simulink model "ornek_6_2"  (R2023b)
settings: Solver=FixedStepDiscrete  StartTime=0.0  StopTime=10  FixedStep=0.1  RelTol=1e-3  EnableMultiTasking=on
undefined symbols (not defined in the file): Timer
libraries: MCHP_Blockset x5, simulink_extras x1
settings Model: Creator=bugra  LastModifiedBy=bugra
settings OptimizationCC: DefaultParameterBehavior=Inlined  DefaultUnderspecifiedDataType=single  EnhancedBackFolding=on  BooleansAsBitfields=on  PassReuseOutputArgsAs=Individual arguments  ZeroExternalMemoryAtStartup=off  ZeroInternalMemoryAtStartup=off  OptimizeBlockOrder=speed  DifferentSizesBufferReuse=on  EfficientTunableParamExpr=on
settings DebuggingCC: ParameterTunabilityLossMsg=error
settings HardwareCC: ProdBitPerInt=16  ProdBitPerPointer=16  ProdBitPerSizeT=16  ProdBitPerPtrDiffT=32  ProdLargestAtomicInteger=Integer  ProdLargestAtomicFloat=None  ProdWordSize=16  ProdHWDeviceType=Generic->Custom
settings ModelReferenceCC: ModelReferenceNumInstancesAllowed=Single
settings SFSimCC: MATLABDynamicMemAlloc=off
settings RTWCC: Description=Microchip Embedded Target PIC24 dsPIC30 dsPIC33 (real-time)  SystemTargetFile=MCHP_dsPIC_stf.tlc  TemplateMakefile=MCHP_dsPIC.tmf
settings CodeAppCC: ForceParamTrailComments=on  IgnoreCustomStorageClasses=off  MaxIdLength=255  OperatorAnnotations=on  SimulinkDataObjDesc=on  SFDataObjDesc=on  InsertBlockDesc=on
settings STFCustomTargetCC: TargetLibSuffix=_lib.a  MultiwordLength=256  CombineOutputUpdateFcns=on  CombineSignalStateStructs=on  SuppressErrorStatus=on  ERTCustomFileBanners=on  SupportContinuousTime=off  RemoveResetFunc=on  MATLABClassNameForMDSCustomization=Simulink.SoftwareTarget.ERTCustomization  SystemTargetFile=MCHP_dsPIC_stf.tlc
settings ERTTargetCC: TargetLibSuffix=_lib.a  TargetLangStandard=C99 (ISO)  ParMdlRefBuildCompliant=off  CompOptLevelCompliant=off  ConcurrentExecutionCompliant=off  CombineSignalStateStructs=on  SuppressErrorStatus=on  SupportNonInlinedSFcns=on  ModelStepFunctionPrototypeControlCompliant=off  CPPClassGenCompliant=off  UseToolchainInfoCompliant=off  ExtModeStaticAllocSize=500  InlinedParameterPlacement=NonHierarchical  ERTSrcFileBannerTemplate=MCHP_dsPIC_code_template.cgt  ERTHdrFileBannerTemplate=MCHP_dsPIC_code_template.cgt  ERTDataSrcFileTemplate=MCHP_dsPIC_code_template.cgt  ERTDataHdrFileTemplate=MCHP_dsPIC_code_template.cgt  ERTCustomFileTemplate=MCHP_main.tlc  MaxLineWidth=110

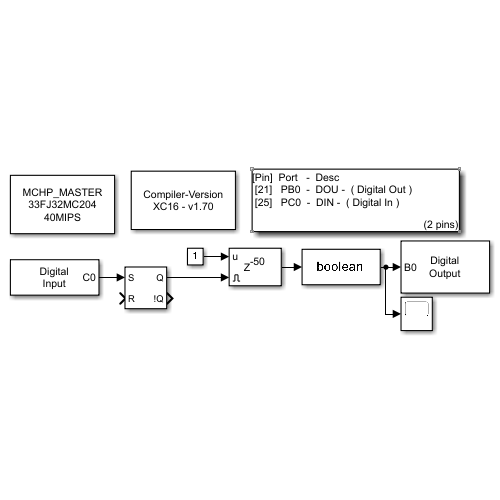
[thumbnail: Simulink's stored preview of the top-level diagram]
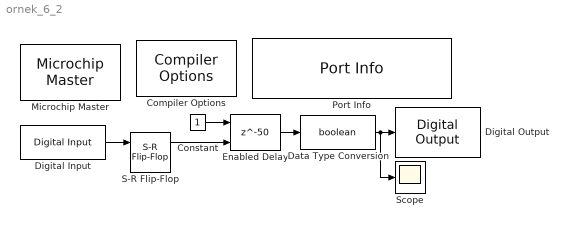
== system ornek_6_2 ==
  Compiler Options : MCHP_Blockset/System Configuration/Compiler Options  Priority=1  LATEST_CMPLR=off  COMP_LIST_TXT=XC16 - v1.70  DFP_LIST_TXT=v 1.4.235  CMSIS_DSP_TXT=Dynamic Options  USE_64BIT_DOUBLE=off  MCHP_MULTITHREAD_COMPILATION=on  UseCustom_LinkerScript=off  MCHP_MASTERLINK=ornek_6_2/Microchip Master  OPTIMIZATION_LEVEL=2  MPLAB_LINKLIB=default  MPLAB_LINKLIB1=fast floating-point math  CodeReplacement_TXT=None  OPTIMIZATION_FLTO=off  OPTIMIZATION_REORDER=off  OPTIMIZATION_ASM_REORDER=off  UNROLL_LOOPS=off  PROCEDURAL_ABSTRACTION=off  GC_SECTIONS=None  MCODE=is less than 32768 (faster)  MCONST=in data memory  MDATA=Use only memory below address 8192 (faster)  MSCALAR=Use only memory below address 8192 (faster)  MLARGEARRAY=off  MAGGREGATE=off  HEAP_SIZE=0  OMF=elf  DEBUG_INFO=off  MCHP_STACK_USAGE=off  GCC_STACK_USAGE=off  ProduceHexOutput=on  AssemblyListing=off  SaveTemps=off  NO_EDS_WARN=on  PRINT_STATISTICS=off
      settings: SourceProductName=MPLAB Device Blocks for Simulink
  Constant : Constant
  Data Type Conversion : DataTypeConversion  OutDataTypeStr=boolean  SaturateOnIntegerOverflow=off  RndMeth=Floor
  Digital Input : MCHP_Blockset/Digital IO/Digital Input  PORT_TXT="C   [ 0 : 9 ]"  PIN=[0]  INPUT_PIN_MODE=Hi-impedance (default)  PACK=off  SIMULTANEOUS=off  ORDERING=None  SampleTime=-1  MCHP_PORT={Digital In}{DIN}2:0:C0;  MCHP_MASTERLINK=ornek_6_2/Microchip Master
      settings: SourceProductName=MPLAB Device Blocks for Simulink
  Digital Output : MCHP_Blockset/Digital IO/Digital Output  PORT=Dynamic Options  PORT_TXT="B   [ 0 : 15 ]"  PIN=0  INIT_VALUE=-1  PACK=off  OUTPUT_PIN_MODE=Push-Pull (default)  SIMULTANEOUS=off  READPREVIOUS=off  ORDERING=None  SampleTime=-1  MCHP_MASTERLINK=ornek_6_2/Microchip Master
      settings: SourceProductName=MPLAB Device Blocks for Simulink
  Enabled Delay : Delay  DelayLength=50  ShowEnablePort=on
      settings: InputPortMap=u0,e6
  Microchip Master : MCHP_Blockset/System Configuration/Microchip Master  Priority=1  PICREF=33FJ32MC204  TIMESTEP_REF="Timer  ( 0.1s )"  BUSYFLAG=Dynamic Options  BUSYFLAG_TXT=None  VDD_range=Dynamic Options  PWRTEN=Not used  BOREN=Enabled  BODENV=2.7V  BORV=Not used  FPWRT=128ms  DSBOREN=Disable ZPBOR during Deep Sleep Mode  DSLPBOR=Not used  MCLRE=Enabled  SMCLR=MCLR pin generates a normal system Reset  PMDL1WAY=Allow only one reconfiguration  RSTPRI=Device will obtain reset instruction from Primary flash  TEMP=Not used  SOSCSRC=Not used  SOSCSEL=Not used  IOL1WAY=Allow Only One Re-configuration  ALTVREF=Not used  DISUVREG=Not used  DSSWEN=Not used  LPCFG=Not used  RTCBAT=Not used  VBTBOR=Not used  WUTSEL=Not used  POWERSAVE=off  FNOSC=Primary Oscillator (XT; HS; EC)  FPR=ECIO w/ PLL 16x  FOSFPR=HS3 w/PLL 16x  FOS=Primary Oscillator  FRANGE=High Range  OSCILLATOR_SELECT=Crystal / Ceramic resonator  OSCILLATOR_SELECT_spd=Crystal / Ceramic resonator  QUARTZ=10e6  QUARTZ_spd=10e6  POSCGAIN=2x gain setting  POSCBOOST=Boost the kick start of the oscillator  SOSCGAIN=2x gain setting  SOSCBOOST=Boost the kick start of the oscillator  ACTIV_PLL=on  ACTIV_PLL_spd=on  MIPS_DESIRED=40000000  MIPS_DESIRED_spd=40000000  CPUDIV=Divide by 1  FPLLMUL=Not used  FPLLIDIV=8x Divider  POSCFREQ=Not used  POSCMD=HS Oscillator Mode  POSCMOD=Primary osc disabled  MIPS=40 * 1e6  ACLKCON=Optimized for PWM resolution & ADC conversion speed  ACLKCON_spd=Optimized for PWM resolution & ADC conversion speed  FPLLODIV=32x Divider  PLLKEN=Clock switch to PLL source will wait until the PLL lock signal is valid  FCKSM=Clock switching is enabled; Fail-Safe Clock Monitor is Disabled  FCKSMEN=Sw Disabled; Mon Disabled  IESO=Start up with FRC; then switch  DSWDTPS=1:2^36  FWDTEN=Disable  FWDTWINSZ=Window size is 25%  FWPSA=1:512  FWPSA0=1:128  FWPSB=1:16  WDT=Disable  WDTPOST=1:32768  WDTPRE=1:128  WDTPS=1:1048576  WINDIS=Watchdog Timer in Non-Window mode  WWDTEN=Window mode  DSWDTEN=Disable DSWDT during Deep Sleep Mode  DSWDTOSC=Select LPRC as DSWDT Reference clock  FWDT_RCLKSEL=WDT Run Mode uses BFRC:256  FWDT_RWDTPS=1:2147483648  FWDT_SWDTMPS=1:2147483648  FWDT_WDTEN=Enable  FWDT_WDTRSTEN=WDT event generates a reset  FWDT_WDTWIN=WDT Window is 25% of WDT period  FWDT_WINEN=Not used  FPBDIV=Not used  FSOSCEN=Disable Secondary Oscillator  LPRCSEL=Not used  OSCIOFCN=Not used  OSCIOFNC=general purpose digital I/O pin  LVRCFG=Not used  PLL_96MHZ=Not used  PLL96MHZ=Not used  PLLDIV=Not used  WDTCLK=Not used  WDTCMX=Not used  WDTWIN=Watchdog Window is 25% of WDT period  XTCFG=24-32 MHz crystals  XTBST=Boost the kick-start  APL=Aux Flash Code protect is disabled  APLK=Aux Flash Write Protection or Code Protection is Enabled  AWRP=Auxiliary program memory is not write-protected  BSS=No Boot program Flash segment  BWP=Not used  BWRP=Boot Segment may be written  CP=Protection Disabled  EBS=No Boot EEPROM  ESS=No Segment Data EEPROM  GCP=General Segment Code protect is Disabled  GSS=High Security Code Protection Enabled  GSS0=Not used  GSSK=General Segment Write Protection or Code Protection is Enabled  GWRP=General Segment may be written  PWP=Not used  RBS=No Boot RAM  RSS=No Secure RAM  SSS=No Secure Segment  SWRP=Secure segment may be written  WPCFG=Not used  WPDIS=Not used  WPEND=Not used  WPFP=Not used  ICESEL=Communicate on PGEC1/PGED1  ICS=Communicate on PGEC1 and PGED1  JTAGEN=Disable  FICD_JTAGEN=Disable  COE=Not used  RES=Not used  DEBUG=Debugger is disabled  BACKBUG=Not used  BKBUG=Not used  ALTI2C=I2C mapped to SDA1/SCL1 pins  ALTI2C1=SDA1/SCK1 pins are selected as the I/O pins for I2C1  ALTI2C2=SDA2/SCK2 pins are selected as the I/O pins for I2C2  ALTI2C3=I2C3 mapped to SDA3/SCL3 pins  FDEVOPT1_ALTI2C1=Not used  FDEVOPT1_ALTI2C2=Not used  FDEVOPT1_SPI2MAPDIS=Not used  FDEVOPT_ALTI2C1=Primary I2C1 pins are used  FDEVOPT_ALTI2C2=Primary I2C2 pins are used  FDEVOPT_ALTI2C3=Primary I2C3 pins are used  FDEVOPT_SPI2PIN=SPI2 pins are selected by peripheral pin selection feature  ALTQIO=QEA1; QEB1; INDX1 are selected as inputs to QEI1  ALTSS1=SS1A is selected as the I/O pin for SPI1  CMPPOL0=Hysteresis is applied to falling edge  CMPPOL1=Hysteresis is applied to falling edge  FCANIO=Not used  FETHIO=Default Ethernet I/O  FMIIEN=MII Enabled  FSRSSEL=Not used  FUSBIDIO=Controlled by the USB Module  FVBUSONIO=Not used  HPOL=PWM module high side output pins have active-high output polarity  HYST0=45 mV Hysteresis  HYST1=45 mV Hysteresis  I2C1SEL=Not used  LPOL=PWM module low side output pins have active-high output polarity  PWMPIN=PWM module pins controlled by PORT register at device Reset  RTCOSC=Not used  UPLLEN=USB PLL Disabled  UPLLIDIV=Not used  ATMOD8=Not used  ALTPMP=Not used  I2C2SEL=Not used  ALTADREF=Not used  ALTCVREF=Not used  PWMLOCK=PWM registers may be written without key sequence  INT_PRIORITY_DMA=0  MCHP_TIMER_REQUEST={Time Step}{TS}0:2:3:1:[]:4000000;  MCHP_TIMER_RESULT=[1 62498.999999999992724 ]  MCHP_PLLRegisters="[5    110  16385     -1     -1]"  MCHPVAR=MCHP.fcy.MIPS=40000000;MCHP.fcy.SYSCLK=40000000;MCHP.fcy.ADC=40000000;MCHP.fcy.Comparator=40000000;MCHP.fcy.I2C=40000000;MCHP.fcy.SPI=40000000;MCHP.fcy.UART=40000000;MCHP.fcy.Timers=40000000;MCHP.fcy.OC=40000000;MCHP.fcy.IC=40000000;MCHP.fcy.Ports=40000000;MCHP.fcy.QEI=40000000;MCHP.PowerSave=0;MCHP.TimeStepFactor=MCHP_Fun.Hex2num('3FF0000000000001');MCHP.TimeStep_Timer=1;MCHP.NTIMERS=3;MCHP.id.name='33FJ32MC204';MCHP.id.N=reshape([33 32 204],1,3);MCHP.id.L=reshape({ 'FJ','MC',''},1,3);MCHP.id.Arch=3;MCHP.id.maskset='';MCHP.id.dos='00899';MCHP.id.ds='70000283';MCHP.id.archTxt='33xxxx';MCHP.id.clonedfrom='DSPIC33FJ32MC204';MCHP.id.isSlave=0;MCHP.id.isMaster=0;MCHP.periph.PPS.reg_RPINRx=reshape([-1 1 1 -1 -1 -1 1 1 -1 -1 -1 -1 -1 -1 1 1 -1 -1 -1 -1 1 1 -1 -1 1 -1 1 -1 1 1 1 -1 -1 -1 -1 -1 1 1 -1 -1 1 1 1],1,43);MCHP.periph.pin.ODCx=reshape([1951 65535 1023 0 0 0 0 0 0 0 0],1,11);MCHP.PPS.dsPIC.RP=reshape([16 17 18 19 20 21 22 23 24 25 26 27 28 29 30 31 32 33 34 35 36 37 38 39 40 41],1,26);MCHP.PPS.dsPIC.RPI=[];MCHP.PPS.dsPIC.RPINR_list=reshape({ '1','INT1','INT2','INT3','INT4','T1CK','T2CK','T3CK','T4CK','T5CK','T6CK','T7CK','T8CK','T9CK','IC1','IC2','IC3','IC4','IC5','IC6','IC7','IC8','OCFA','OCFB','FLT1','FLT2','FLT3','FLT4','QEIA1','QEIB1','QEINDX1','QEIHOM1','QEIA2','QEIB2','QEINDX2','QEIHOM2','U1RX','U1CTS','U2RX','U2CTS','SDI1','SCK1_in','SS1_in','44','SDI2','SCK2_in','SS2_in','48','CSDIR','CSCK','COFS','52','C1RX','C2RX','U3RX','U3CTS','U4RX','U4CTS','SDI3','SCK3_in','SS3_in','62','SDI4','SCK4_in','SS4_in','66','IC9','IC10','IC11','IC12','IC13','IC14','IC15','IC16','OCFC','SYNCI1','SYNCI2','DTCMP1','DTCMP2','DTCMP3','DTCMP4','DTCMP5','DTCMP6','DTCMP7','FLT5','FLT6','FLT7','FLT8','89','SENT1','SENT2','92'},1,92);MCHP.PPS.dsPIC.RPOR_list=reshape({ '1','C1OUT','C2OUT','U1TX','U1RTS','U2TX','U2RTS','SDO1','SCK1_out','SS1_out','SDO2','SCK2_out','SS2_out','CSDO','CSCK','COFS','C1TX','17','OC1','OC2','OC3','OC4','22','23','24','25','UPDN1','UPDN2'},1,28);MCHP.PPS.dsPIC.RPV=reshape([-1 -1 -1 -1 -1 -1],1,6);MCHP.PPS.map_RPnR_RPORx=reshape([0 1 2 3 4 5 6 7 8 9 10 11 12 13 14 15 16 17 18 19 20 21 22 23 24 25],1,26);MCHP.Rx=reshape([19 21 25 -1 -1 -1 -1 -1 -1 -1 -1 20 22 26 -1 -1 -1 -1 -1 -1 -1 -1 30 23 27 -1 -1 -1 -1 -1 -1 -1 -1 31 24 36 -1 -1 -1 -1 -1 -1 -1 -1 34 33 37 -1 -1 -1 -1 -1 -1 -1 -1 -1 41 38 -1 -1 -1 -1 -1 -1 -1 -1 -1 42 2 -1 -1 -1 -1 -1 -1 -1 -1 13 43 3 -1 -1 -1 -1 -1 -1 -1 -1 32 44 4 -1 -1 -1 -1 -1 -1 -1 -1 35 1 5 -1 -1 -1 -1 -1 -1 -1 -1 12 8 -1 -1 -1 -1 -1 -1 -1 -1 -1 -1 9 -1 -1 -1 -1 -1 -1 -1 -1 -1 -1 10 -1 -1 -1 -1 -1 -1 -1 -1 -1 -1 11 -1 -1 -1 -1 -1 -1 -1 -1 -1 -1 14 -1 -1 -1 -1 -1 -1 -1 -1 -1 -1 15 -1 -1 -1 -1 -1 -1 -1 -1 -1],11,16);MCHP.ADC.ANtype=reshape([3 0],1,2);MCHP.ADC.ADCONx=reshape([59375 59327 40959 0 0 0],1,6);MCHP.ADC.ADCHS_0=reshape([40863 1799],1,2);MCHP.ADC.Flags=reshape([1 0],1,2);MCHP.ADC.Buffer=reshape([16 -1],1,2);MCHP.ADC.port=reshape([0 1 16 17 18 19 32 33 34 -1 -1 -1 -1 -1 -1 -1 -1 -1 -1 -1 -1 -1 -1 -1 -1 -1 -1 -1 -1 -1 -1 -1 -1 -1 -1 -1 -1 -1 -1 -1 -1 -1 -1 -1 -1 -1 -1 -1 -1 -1 -1 -1 -1 -1 -1 -1 -1],1,57);MCHP.ADC.port_ALT=reshape([-1 -1 -1 -1],1,4);MCHP.ADC.port_ALTA=reshape([-1 -1 -1 -1],1,4);MCHP.ADC.port_ALTB=reshape([-1 -1 -1 -1],1,4);MCHP.ADC.port_ALTC=reshape([-1 -1 -1 -1],1,4);MCHP.ADC.port_VrefP=0;MCHP.ADC.port_VrefM=1;MCHP.ADC.port_AVdd=-1;MCHP.ADC.port_AVss=-1;MCHP.ADC.ADCDATA=reshape([0 0 0 0 0 0 0 0 0 0 0 0 0 0 0 0 0 0 0 0 0 0 0 0 0 0 0 0 0 0 0 0 0 0 0 0 0 0 0 0 0 0 0 0 0 0 0 0 0 0 0 0 0 0 0 0 0],1,57);MCHP.ADC.HS_SAR.TRGSRC=reshape([0 0 0 0 0 0 0 0 0 0 0 0 0 0 0 0 0 0 0 0 0 0 0 0 0 0 0 0 0 0 0 0],1,32);MCHP.ADC.HS_SAR.nFilters=0;MCHP.ADC.HS_SAR.nDedicatedCore=0;MCHP.ADC.HS_SAR.CALIBRATION=0;MCHP.ADC.HS_SAR.ADCON1L=-1;MCHP.ADC.HS_SAR.ADC_Class3_idxStart=32;MCHP.memory.RAM=2048;MCHP.memory.RAM_XBegin=2048;MCHP.memory.RAM_YBegin=3072;MCHP.memory.RAM_dma=reshape([-1 -1],1,2);MCHP.memory.FLASH_ECC=0;MCHP.DMA.Num=0;MCHP.DMA.CNTmax=0;MCHP.QEI.QEICONx=reshape([49151 -1 -1 -1 -1 -1],1,6);MCHP.QEI.QEItype=1;MCHP.QEI.Port_QEI_INDX=reshape([-1 -1],1,2);MCHP.QEI.Port_QEI_QEA=reshape([-1 -1],1,2);MCHP.QEI.Port_QEI_QEB=reshape([-1 -1],1,2);MCHP.QEI.Port_QEI_UPDN=reshape([-1 -1],1,2);MCHP.INT.Port=reshape([23 32767 32767 -1 -1],1,5);MCHP.ADC1.port=reshape([-1 -1 -1 -1 -1 -1 -1 -1 -1 -1 -1 -1 -1 -1 -1 -1 -1 -1 -1 -1 -1 -1 -1 -1 -1 -1 -1 -1 -1 -1 -1 -1],1,32);MCHP.ADC2.port=reshape([-1 -1 -1 -1 -1 -1 -1 -1 -1 -1 -1 -1 -1 -1 -1 -1 -1 -1 -1 -1 -1 -1 -1 -1 -1 -1 -1 -1 -1 -1 -1 -1],1,32);MCHP.ADC3.port=reshape([-1 -1 -1 -1 -1 -1 -1 -1 -1 -1 -1 -1 -1 -1 -1 -1],1,16);MCHP.ADC4.port=reshape([-1 -1 -1 -1 -1 -1 -1 -1 -1 -1 -1 -1 -1 -1 -1 -1],1,16);MCHP.ADC5.port=reshape([-1 -1 -1 -1 -1 -1 -1 -1 -1 -1 -1 -1 -1 -1 -1 -1],1,16);MCHP.ADC1N.port=reshape([-1 -1 -1 -1],1,4);MCHP.ADC2N.port=reshape([-1 -1 -1 -1],1,4);MCHP.ADC3N.port=reshape([-1 -1 -1 -1],1,4);MCHP.ADC4N.port=reshape([-1 -1 -1 -1],1,4);MCHP.ADC5N.port=reshape([-1 -1 -1 -1],1,4);MCHP.PWM_HS.Flags=reshape([0 0 0],1,3);MCHP.PWM.port_FLT=reshape([-1 -1 -1 -1 -1 -1 -1 -1 -1 -1 -1 -1 -1 -1 -1 -1 -1 -1 -1 -1 -1 -1 -1 -1 -1 -1 -1 -1 -1 -1 -1 -1 -1],1,33);MCHP.PWM.PWMRef=2;MCHP.PWM.Flag=2;MCHP.PWM.Port_PWM_l=reshape([31 39 29 -1 27 -1 -1 -1 -1 -1 -1 -1 -1 -1 -1 -1 -1 -1 -1 -1 -1 -1 -1 -1],2,12);MCHP.PWM.Port_PWM_h=reshape([30 38 28 -1 26 -1 -1 -1 -1 -1 -1 -1 -1 -1 -1 -1 -1 -1 -1 -1 -1 -1 -1 -1],2,12);MCHP.PWM_HS_FEP.nEVTOUT=-1;MCHP.IC.Port=reshape([32767 32767 0 0 0 0 32767 32767 0 0 0 0 0 0 0 0],1,16);MCHP.IC.type=0;MCHP.OC.Port=reshape([32767 32767 0 0 0 0 32767 32767 0 0 0 0 0 0 0 0],1,16);MCHP.OC.type=0;MCHP.CN.Port=reshape([4 20 0 1 16 17 18 19 32 33 34 31 30 29 28 27 26 39 38 41 40 25 24 23 22 36 37 21 35 3 2 -1 -1 -1 -1 -1 -1 -1 -1 -1 -1 -1 -1 -1 -1 -1 -1 -1 -1 -1 -1 -1 -1 -1 -1 -1 -1 -1 -1 -1 -1 -1 -1 -1 -1 -1 -1 -1 -1 -1 -1 -1 -1 -1 -1 -1 -1 -1 -1 -1 -1 -1 -1 -1 -1],1,85);MCHP.CN.PullUp=reshape([65535 32767 0 0 0 0 0 0 0 0 0],1,11);MCHP.CN.type=0;MCHP.CN.Flag_PullDown=1;MCHP.SPI.Refs=reshape([1 0 0 0 0 0],1,6);MCHP.SPI.SPIxCON1=8191;MCHP.SPI.SPIxCON2=57346;MCHP.SPI.SPIxFIFOSIZE=-1;MCHP.SPI.Port_SDI=reshape([-1 -1 -1 -1 -1 -1],1,6);MCHP.SPI.Port_SDO=reshape([-1 -1 -1 -1 -1 -1],1,6);MCHP.SPI.Port_SCK=reshape([-1 -1 -1 -1 -1 -1],1,6);MCHP.SPI.Port_SS=reshape([-1 -1 -1 -1 -1 -1],1,6);MCHP.I2C.Refs=reshape([1 0 0 0 0],1,5);MCHP.I2C.I2CxCON=65535;MCHP.I2C.NewRegName=1;MCHP.I2C.Port_SDA=reshape([25 -1 -1 -1 -1],1,5);MCHP.I2C.Port_SCL=reshape([24 -1 -1 -1 -1],1,5);MCHP.I2C.Port_ASDA=reshape([21 -1 -1 -1 -1],1,5);MCHP.I2C.Port_ASCL=reshape([22 -1 -1 -1 -1],1,5);MCHP.I2C.Fuse_Port_SCL_SDA=reshape([16 1 -1 -1 -1 -1 -1 -1 -1 -1],2,5);MCHP.I2C.Fuse_Port_ASCL_ASDA=reshape([16 2 -1 -1 -1 -1 -1 -1 -1 -1],2,5);MCHP.SCCP.nSCCP=0;MCHP.SCCP.MCCP=reshape([0 0 0 0 0 0 0 0 0],1,9);MCHP.PGA.Port_PGA1P=reshape([-1 -1 -1 -1],1,4);MCHP.PGA.Port_PGA1N=reshape([-1 -1 -1 -1],1,4);MCHP.PGA.Port_PGA2P=reshape([-1 -1 -1 -1],1,4);MCHP.PGA.Port_PGA2N=reshape([-1 -1 -1 -1],1,4);MCHP.PGA.Num=0;MCHP.HS_AnalogComparator.Port_CMP1=reshape([-1 -1 -1 -1],1,4);MCHP.HS_AnalogComparator.Port_CMP2=reshape([-1 -1 -1 -1],1,4);MCHP.HS_AnalogComparator.Port_CMP3=reshape([-1 -1 -1 -1],1,4);MCHP.HS_AnalogComparator.Port_CMP4=reshape([-1 -1 -1 -1],1,4);MCHP.HS_AnalogComparator.Port_CMP5=reshape([-1 -1 -1 -1],1,4);MCHP.HS_AnalogComparator.Port_CMP6=reshape([-1 -1 -1 -1],1,4);MCHP.HS_AnalogComparator.Port_EXTREFx=reshape([-1 -1],1,2);MCHP.HS_AnalogComparator.Port_DACOUTx=reshape([-1 -1],1,2);MCHP.HS_AnalogComparator.Num=0;MCHP.Comp.Port_CVrefin=-1;MCHP.Comp.Port_CVref=-1;MCHP.Comp.Port_CVref1O=-1;MCHP.Comp.Port_CVref2O=-1;MCHP.Comp.Port_CxOUT=reshape([32767 32767 32767 32767 32767],1,5);MCHP.Comp.Port_OAxOUT=reshape([-1 -1 -1 -1 -1],1,5);MCHP.Comp.Port_CxINP=reshape([-1 17 -1 -1 -1],1,5);MCHP.Comp.Port_CxINM=reshape([-1 -1 -1 -1 16 -1 -1 -1 -1 -1 -1 -1 -1 -1 -1 -1 -1 -1 -1 -1],4,5);MCHP.Comp.Port_OAxINP=reshape([-1 -1 -1 -1 -1],1,5);MCHP.Comp.Port_OAxINM=reshape([-1 -1 -1 -1 -1],1,5);MCHP.Comp.nComp=reshape([5 0 0],1,3);MCHP.Comp.OpAmp=0;MCHP.Comp.CVRCON=reshape([0 0],1,2);MCHP.Comp.CMCON=0;MCHP.CDAC.Port_DACx=reshape([-1 -1 -1],1,3);MCHP.CDAC.nCDAC=0;MCHP.UART.port_Rx=reshape([32767 -1 -1 -1 -1 -1],1,6);MCHP.UART.port_Tx=reshape([32767 -1 -1 -1 -1 -1],1,6);MCHP.UART.port_ARx=reshape([-1 -1],1,2);MCHP.UART.port_ATx=reshape([-1 -1],1,2);MCHP.UART.port_RTS=reshape([32767 -1 -1 -1 -1 -1],1,6);MCHP.UART.port_CTS=reshape([32767 -1 -1 -1 -1 -1],1,6);MCHP.UART.reg_UxMODE=reshape([48127 -1 -1 -1 -1 -1],1,6);MCHP.UART.reg_UxSTA=reshape([61439 -1 -1 -1 -1 -1],1,6);MCHP.modsrc.DOS_04094_cpu_33a_v1_dspic33a=0;MCHP.modsrc.DOS_04436_perseus_dspic33a=0;MCHP.modsrc.DOS_04928_gpio_ports_upb_v2_dspic33a=0;MCHP.modsrc.DOS_02672_math_progcrc_upb_v1_dspic33a=0;MCHP.modsrc.DOS_04993_sec_32bit_cp_upb_v1_dspic33a=0;MCHP.modsrc.DOS_03681_bmx_33a_upb_v1_dspic33a=0;MCHP.modsrc.DOS_03459_adc_pc_ctrl_upb_v2_dspic33a=0;MCHP.modsrc.DOS_04302_pwm_pc_upb_v3_dspic33a=0;MCHP.modsrc.DOS_03076_uart_protocol_upb_v1_dspic33a=0;MCHP.modsrc.DOS_01482_spi_i2s_upb_v1_dspic33a=0;MCHP.modsrc.DOS_05155_i2c_upb_v4_dspic33a=0;MCHP.modsrc.DOS_02359_sent_j2716_upb_v1_dspic33a=0;MCHP.modsrc.DOS_05177_qei_32b_upb_v2_dspic33a=0;MCHP.modsrc.DOS_01512_ccp_mccp_upb_v1_dspic33a=0;MCHP.modsrc.DOS_03496_dac_pdm_nbit_upb_v2_dspic33a=0;MCHP.modsrc.DOS_02673_tmr_classa_upb_v1_dspic33a=0;MCHP.modsrc.DOS_04776_perf_mon_upb_v1_dspic33a=0;MCHP.modsrc.DOS_03680_pfm_pbu_33a_upb_v1_dspic33a=0;MCHP.modsrc.DOS_04649_sec_pac_upb_v0_dspic33a=0;MCHP.modsrc.DOS_03966_io_integrity_monitor_upb_v1_dspic33a=0;MCHP.modsrc.DOS_04641_biss_master_upb_v1_dspic33a=0;MCHP.modsrc.DOS_04077_dma_upb_v1_dspic33a=0;MCHP.modsrc.DOS_04549_nvm_ctrl_32bit_upb_v1_dspic33a=0;MCHP.modsrc.DOS_04449_clk_cru_33a_upb_v1_dspic33a=0;MCHP.modsrc.DOS_03850_clk_monitor_upb_v1_dspic33a=0;MCHP.modsrc.DOS_04342_osc_rc8mhz_ctrl_upb_v4_dspic33a=0;MCHP.modsrc.DOS_04650_wdt_upb_v4_dspic33a=0;MCHP.modsrc.DOS_05178_ptg_pc_upb_v1_dspic33a=0;MCHP.modsrc.DOS_04181_data_ram_ctrl_upb_v1_dspic33a=0;MCHP.modsrc.DOS_04735_wdt_dmt_upb_v6_dspic33a=0;MCHP.modsrc.DOS_01577_cla_clc_upb_v1_dspic33a=0;MCHP.modsrc.DOS_03516_pwr_sib_upb_v3_dspic33a=0;MCHP.modsrc.DOS_03495_amp_pad_opamp_ctrl_upb_v2_dspic33a=0;MCHP.modsrc.DOS_05308_pegasus_dspic33a=0;MCHP.modsrc.DOS_02976_adc_12b_upb_v2_dspic33a=0;MCHP.modsrc.DOS_05404_adc_pc_ctrl_upb_v3_dspic33a=0;MCHP.modsrc.DOS_05226_pwm_pc_upb_v4_dspic33a=0;MCHP.modsrc.DOS_05226_apwm_pc_upb_v4_dspic33a=0;MCHP.modsrc.DOS_05431_dac_pdm_nbit_upb_v3_dspic33a=0;MCHP.modsrc.DOS_04649_sec_pac_upb_v1_dspic33a=0;MCHP.modsrc.DOS_05461_pwr_sib_upb_v4_dspic33a=0;MCHP.modsrc.DOS_05420_amp_vref_ctl_upb_v1_dspic33a=0;MCHP.modsrc.DOS_03267_adc_soft_code_seq_v1_dspic33a=0;MCHP.modsrc.DOS_04537_can_fd_upb_v3_dspic33a=0;MCHP.modsrc.DOS_05346_sec_cam_lite_v2_dspic33a=0;MCHP.modsrc.DOS_05830_blueRidge_dspic33a=0;MCHP.modsrc.DOS_05765_math_rdc_upb_v1_32bit=0;MCHP.modsrc.DOS_05908_math_cic_upb_v2_32bit=0;MCHP.modsrc.DOS_05922_i3c_upb_v1_32bit=0;MCHP.modsrc.DOS_05442_icd_trace_33a_v1_dspic33a=0;MCHP.modsrc.DOS_02551_cpu_16bit_v7=0;MCHP.modsrc.DOS_01520_wdt_dmt_upb_v1_16bit=0;MCHP.modsrc.DOS_02359a_sent_j2716_upb_v1=0;MCHP.modsrc.DOS_02672_math_progcrc_upb_v1_16bit=0;MCHP.modsrc.DOS_01577_cla_clc_upb_v1=0;MCHP.modsrc.DOS_02915_ecc_v2=0;MCHP.modsrc.DOS_02673_tmr_classa_upb_v1_16bit=0;MCHP.modsrc.DOS_01494_qei_32b_upb_v1_16bit=0;MCHP.modsrc.DOS_02472_ppi_pmp16_upb_v1_16bit=0;MCHP.modsrc.DOS_01441_i2c_upb_v1_16bit_TLAH=0;MCHP.modsrc.DOS_03076_uart_protocol_upb_v1_16bit=0;MCHP.modsrc.DOS_01482=0;MCHP.modsrc.DOS_01483_pwm_16bit=0;MCHP.modsrc.DOS_02949_WACG=0;MCHP.modsrc.DOS_02316_nvm_ctrl_v1_16bit=0;MCHP.modsrc.DOS_03349_amp_pad_opamp_ctrl_upb_v1=0;MCHP.modsrc.DOS_02653_afe_current_bias_ctrl_upb_v1_16bit=0;MCHP.modsrc.DOS_01459_ptg_pc_upb_v1_16bit=0;MCHP.modsrc.DOS_01512_ccp_mccp_upb_v1_16bit=0;MCHP.modsrc.DOS_02519_dma_sfr_16bit_v2=0;MCHP.modsrc.DOS_02508c11=0;MCHP.modsrc.DOS_02475_dac_pdm_nbit_upb_v1_16bit=0;MCHP.modsrc.DOS_02467_gpio_upb_v1_16bit=0;MCHP.modsrc.DOS_00805_rst_integration_v4=0;MCHP.modsrc.DOS_02659_clk_sib_v12=0;MCHP.modsrc.DOS_02237_osc_dco_ctrl_upb_v1_16bit=0;MCHP.modsrc.DOS_02674_wdt_upb_v1_16bit=0;MCHP.modsrc.DOS_01407=0;MCHP.modsrc.DOS_03247_CAN_FD_UPB_V2_16_bit=0;MCHP.modsrc.DOS_03994_WAC07=0;MCHP.modsrc.DOS_02552_msi_upb_v1_Master=0;MCHP.modsrc.DOS_03667_pwm_pc_upb_v2_16bit=0;MCHP.modsrc.DOS_04180_drm_ctrl_ecc_v1=0;MCHP.modsrc.DOS_03431_STX03=0;MCHP.modsrc.DOS_03516_pwr_sib_upb_v3=0;MCHP.modsrc.DOS_02552_msi_upb_v1_Slave=0;MCHP.modsrc.DOS_04621_amp_pga_ctrl_upb_v3=0;MCHP.modsrc.DOS_02497_WACV=0;MCHP.modsrc.DOS_02593_amp_pga_ctrl_pb_v2_16bit=0;MCHP.modsrc.DOS_01461_afe_ctmu_con_upb_v1_16bit=0;MCHP.modsrc.DOS_02497_WACA=0;MCHP.modsrc.DOS_02478_uart_irda_upb_v1_16bit=0;MCHP.modsrc.DOS_00929=0;MCHP.modsrc.DOS_01198=0;MCHP.modsrc.DOS_03029_WACH=0;MCHP.modsrc.DOS_01483_apwm_16bit=0;MCHP.modsrc.DOS_04797_WAC0A=0;MCHP.modsrc.DOS_04884_WAC0B=0;MCHP.modsrc.DOS_04797_WAC09=0;MCHP.modsrc.DOS_03662_WACU=0;MCHP.modsrc.DOS_00794=0;MCHP.modsrc.DOS_00931=0;MCHP.modsrc.DOS_00932=0;MCHP.modsrc.DOS_00942=0;MCHP.modsrc.DOS_00938=0;MCHP.modsrc.DOS_00996=0;MCHP.modsrc.DOS_00997=0;MCHP.modsrc.DOS_00998=0;MCHP.modsrc.DOS_00209=0;MCHP.modsrc.DOS_01555_adc=0;MCHP.modsrc.DOS_01293=0;MCHP.modsrc.DOS_00828=0;MCHP.modsrc.DOS_01116=0;MCHP.modsrc.DOS_01017_RPORx=0;MCHP.modsrc.DOS_01017_RPINRx=0;MCHP.modsrc.DOS_01555_nvm_tsmc18_v2_16bit=0;MCHP.modsrc.DOS_00804=0;MCHP.modsrc.DOS_00826=0;MCHP.modsrc.DOS_01555_TLAK_PMDx=0;MCHP.modsrc.DOS_01555_TLAK_INT_=0;MCHP.modsrc.DOS_00933=0;MCHP.modsrc.DOS_01555=0;MCHP.modsrc.DOS_01555_ptg=0;MCHP.modsrc.DOS_00958=0;MCHP.modsrc.DOS_01117_PORTx=0;MCHP.modsrc.DOS_00999=0;MCHP.modsrc.DOS_01041=0;MCHP.modsrc.DOS_00892=0;MCHP.modsrc.DOS_01287_TLAC_PMDx=0;MCHP.modsrc.DOS_01287_TLAC_INT_=0;MCHP.modsrc.DOS_01424=0;MCHP.modsrc.DOS_01332=0;MCHP.modsrc.DOS_01468_PMBA_current_source=0;MCHP.modsrc.DOS_02291_PGA=0;MCHP.modsrc.DOS_01467_Comparator=0;MCHP.modsrc.DOS_01498_TLAY=0;MCHP.modsrc.DOS_00993_PLL_120MHz=0;MCHP.modsrc.DOS_01332_ptg_pc_v1=0;MCHP.modsrc.DOS_00958_pwm_TLAY=0;MCHP.modsrc.TLAY_IOPorts=0;MCHP.modsrc.DOS_00929q=0;MCHP.modsrc.DOS_02415_spi_v5=0;MCHP.modsrc.DOS_RPINRx_16bit_2=0;MCHP.modsrc.DOS_01497_TLAH_PMDx=0;MCHP.modsrc.DOS_02550_TLAL_INT=0;MCHP.modsrc.DOS_00958_pwm_TLAH=0;MCHP.modsrc.DOS_01287_TLAH_INT_=0;MCHP.modsrc.DOS_01113=0;MCHP.modsrc.DOS_01017_PMDx=0;MCHP.modsrc.DOS_00927=0;MCHP.modsrc.DOS_01080=0;MCHP.modsrc.DOS_00794_cpu_16bit_v3=0;MCHP.modsrc.DOS_02192_TLCD_PMDx=0;MCHP.modsrc.DOS_02192_TLCD_INT_=0;MCHP.modsrc.DOS_02192_cmp=0;MCHP.modsrc.DOS_00958_pwm_TLCD=0;MCHP.modsrc.DOS_02192_PORTx_TLCD=0;MCHP.modsrc.DOS_00936=0;MCHP.modsrc.DOS_00995=0;MCHP.modsrc.DOS_00546=0;MCHP.modsrc.DOS_00474=0;MCHP.modsrc.DOS_02481_WACK_MC_Config=0;MCHP.modsrc.DOS_03088_pfm_cache_ocp_v2_WACK=0;MCHP.modsrc.DOS_02819_pfm_ctrl_32bit_upb_v2=0;MCHP.modsrc.DOS_02674_wdt_upb_v1_32bit=0;MCHP.modsrc.DOS_01520_wdt_dmt_upb_v1=0;MCHP.modsrc.DOS_02869_icd_jtag_bvci_upb_v2=0;MCHP.modsrc.DOS_02823_WACJ_clk_cru_upb_v2=0;MCHP.modsrc.DOS_02823_WACN_clk_cru_upb_v2=0;MCHP.modsrc.DOS_01423_RPINRx=0;MCHP.modsrc.DOS_02481_RPORx=0;MCHP.modsrc.DOS_02511_pwr_sib_upb_v1_32bit=0;MCHP.modsrc.DOS_02907_WACN_GP_int_evic_v3=0;MCHP.modsrc.DOS_01500_dma_bvci_v2=0;MCHP.modsrc.DOS_02141_tmr_classa_pb_v2=0;MCHP.modsrc.DOS_02815_tmr_classb_upb_v1=0;MCHP.modsrc.DOS_00740_icap_pb_v1=0;MCHP.modsrc.DOS_00749_ocmp_pb_v1=0;MCHP.modsrc.DOS_01441_i2c_upb_v1_32bit=0;MCHP.modsrc.DOS_01329_spi_pb_v2=0;MCHP.modsrc.DOS_02478_uart_irda_upb_v1_32bit=0;MCHP.modsrc.DOS_03554_cmp_control_upb_v2_32bit=0;MCHP.modsrc.DOS_01445_dac_nbit__control_upb_v1_32bit=0;MCHP.modsrc.DOS_01461_afe_ctmu_con_upb_v1=0;MCHP.modsrc.DOS_01577_cla_clc_upb_v1_32bit=0;MCHP.modsrc.DOS_02467_gpio_ports_upb_v1=0;MCHP.modsrc.DOS_02508_adc_sar_ctrl_upb_v1_PIC32MK=0;MCHP.modsrc.DOS_01261_tmr_rtcc_pb_v2=0;MCHP.modsrc.DOS_01475_lpwr_deep_sleep_ctrl_v2=0;MCHP.modsrc.DOS_EIP_00136_ssx_v1=0;MCHP.modsrc.DOS_02907_WACN_MC_int_evic_v3=0;MCHP.modsrc.DOS_01477_pwm_mc_upb_v1=0;MCHP.modsrc.DOS_01494_qei_32b_upb_v1=0;MCHP.modsrc.DOS_03247_can_fd_upb_v2_pic32mk=0;MCHP.modsrc.DOS_02907_WACK_MC_int_evic_v3=0;MCHP.modsrc.DOS_02514_dfm_strl_sst_upb_v1=0;MCHP.modsrc.DOS_02472_ppi_pmp16_upb_v1=0;MCHP.modsrc.DOS_02813a_usb_otgcore_pb_v3=0;MCHP.modsrc.DOS_02481_WACJ_MC_Config=0;MCHP.modsrc.DOS_02569_pfm_cache_ocp_v1=0;MCHP.modsrc.DOS_02481_WACJ_MC_int_evic_v3=0;MCHP.modsrc.DOS_01459_ptg_pc_upb_v1_SIC=0;MCHP.modsrc.DOS_01427_cmp_control_upb_v1_32bit=0;MCHP.modsrc.DOS_01152_can_bvci_v1=0;MCHP.modsrc.DOS_02787_WACD_Config=0;MCHP.modsrc.DOS_00800_dac_4bit_ctrl_pb_v1=0;MCHP.modsrc.DOS_01539_icd_jtag_pb_v2=0;MCHP.modsrc.DOS_02823_clk_cru_upb_v2=0;MCHP.modsrc.DOS_01423_RPORx=0;MCHP.modsrc.DOS_02907_WACD_int_evic_v3=0;MCHP.modsrc.DOS_00734_uart_irda_pb_v1=0;MCHP.modsrc.DOS_00687_tmr_classa_pb_v1=0;MCHP.modsrc.DOS_00745_tmr_classb_pb_v1=0;MCHP.modsrc.DOS_02508_adc_sar_ctrl_upb_v1=0;MCHP.modsrc.DOS_00866_cmp_control_pb_v2=0;MCHP.modsrc.DOS_01114_eth_bvci_v1=0;MCHP.modsrc.DOS_02831_usb_clk_rst_v2=0;MCHP.modsrc.DOS_01643_pfm_cache_ahb_v2=0;MCHP.modsrc.DOS_EIP_00206r5_sqi_v2=0;MCHP.modsrc.DOS_EIP_00124_usb_hs_otgcore_v1=0;MCHP.modsrc.DOS_EIP_00218_math_rng_ahbs_v2=0;MCHP.modsrc.DOS_EIP_00109_ebi_v1=0;MCHP.modsrc.DOS_EIP_00158_crypto_v1=0;MCHP.PortBase=16;MCHP.PortPrefixe='P';MCHP.clock.PBxDIV=-1;MCHP.clock.CLKx_INTDIV=reshape([-1 -1 -1 -1 -1 -1 -1 -1 -1 -1 -1 -1 -1],1,13);MCHP.clock.CLKx_FRACDIV=reshape([-1 -1 -1 -1 -1 -1 -1 -1 -1 -1 -1 -1 -1],1,13);  MCHP_CRC=20034748  BTMODE=Device is in Single Boot (legacy) mode  RES1=Not used  PLLSS=Not used  RES2=Not used  ALTCMPI=Not used  BOREN1=Not used  ALTRB6=Not used  RETCFG=Not used  DFMCY=Not used  BSS2=No Boot Segment  BSEN=No Boot Segment  CWRP=Configuration Segment may be written  CSS=No Protection (other than CWRP)  AIVTDIS=Disable Alternate Vector Table  BSLIM=Not used  WDTEN=Disable  BTSWP=BOOTSWP instruction is disabled  DBCC=No Cross Connection between DAC outputs  CTXT1=Not Assigned  CTXT2=Not Assigned  SEQNUM=Not used  nSEQNUM=Not used  BOREN0=Enabled  DMTIVT=Not used  DMTCNT=2^8 (256)  DMTEN=Dead Man Timer is Disabled and can be enabled by software  ON=Not used  USERID=Not used  RESERVED1=Not used  PGL1WAY=Allow only one reconfiguration  FPLLRNG=34-68 MHz Input  FPLLICLK=FRC is input to the System PLL  FPLLMULT=PLL Multiply by 128  UPLLFSEL=USB PLL input is 24 MHz  DMTINTV=Window/Interval value is 127/128 counter value  WDTSPGM=WDT stops during Flash programming  FDMTEN=Deadman Timer is disabled  TRCEN=Trace features in the CPU are enabled  BOOTISA=Boot code and Exception code is MIPS32  FECCCON=ECC and Dynamic ECC are disabled (ECCCON bits are writable)  EXTDDRSIZE=Not used  FSLEEP=Flash is powered down when the device is in Sleep mode  DBGPER=Allow CPU access to all permission regions  EJTAGBEN=Normal EJTAG functionality  TSEQ=Not used  CSEQ=Not used  RWDTPS=1:1048576  RCLKSEL=Always use LPRC  SWDTPS=1:1048576  DMTIVTL=Not used  DMTIVTH=Not used  DMTCNTL=Not used  DMTCNTH=Not used  DMTDIS=Dead Man Timer is Disabled and can be enabled by software  SMBEN=SMBus input threshold is enabled  SPI2PIN=SPI2 uses I/O remap (PPS) pins  CTXT3=Not Assigned  CTXT4=Not Assigned  MBXM0=Mailbox register configured for Main data read (Secondary to Main data transfer)  MBXM1=Mailbox register configured for Main data read (Secondary to Main data transfer)  MBXM2=Mailbox register configured for Main data read (Secondary to Main data transfer)  MBXM3=Mailbox register configured for Main data read (Secondary to Main data transfer)  MBXM4=Mailbox register configured for Main data read (Secondary to Main data transfer)  MBXM5=Mailbox register configured for Main data read (Secondary to Main data transfer)  MBXM6=Mailbox register configured for Main data read (Secondary to Main data transfer)  MBXM7=Mailbox register configured for Main data read (Secondary to Main data transfer)  MBXM8=Mailbox register configured for Main data read (Secondary to Main data transfer)  MBXM9=Mailbox register configured for Main data read (Secondary to Main data transfer)  MBXM10=Mailbox register configured for Main data read (Secondary to Main data transfer)  MBXM11=Mailbox register configured for Main data read (Secondary to Main data transfer)  MBXM12=Mailbox register configured for Main data read (Secondary to Main data transfer)  MBXM13=Mailbox register configured for Main data read (Secondary to Main data transfer)  MBXM14=Mailbox register configured for Main data read (Secondary to Main data transfer)  MBXM15=Mailbox register configured for Main data read (Secondary to Main data transfer)  MBXHSA=MSIxMBXD15 assigned to mailbox handshake protocol block A  MBXHSB=MSIxMBXD15 assigned to mailbox handshake protocol block B  MBXHSC=MSIxMBXD15 assigned to mailbox handshake protocol block C  MBXHSD=MSIxMBXD15 assigned to mailbox handshake protocol block D  MBXHSE=MSIxMBXD15 assigned to mailbox handshake protocol block E  MBXHSF=MSIxMBXD15 assigned to mailbox handshake protocol block F  MBXHSG=MSIxMBXD15 assigned to mailbox handshake protocol block G  MBXHSH=MSIxMBXD15 assigned to mailbox handshake protocol block H  HSAEN=Mailbox data flow control handshake protocol block disabled  HSBEN=Mailbox data flow control handshake protocol block disabled  HSCEN=Mailbox data flow control handshake protocol block disabled  HSDEN=Mailbox data flow control handshake protocol block disabled  HSEEN=Mailbox data flow control handshake protocol block disabled  HSFEN=Mailbox data flow control handshake protocol block disabled  HSGEN=Mailbox data flow control handshake protocol block disabled  HSHEN=Mailbox data flow control handshake protocol block disabled  CPRA0=Main core owns pin  CPRA1=Main core owns pin  CPRA2=Main core owns pin  CPRA3=Main core owns pin  CPRA4=Main core owns pin  CPRB0=Main core owns pin  CPRB1=Main core owns pin  CPRB2=Main core owns pin  CPRB3=Main core owns pin  CPRB4=Main core owns pin  CPRB5=Main core owns pin  CPRB6=Main core owns pin  CPRB7=Main core owns pin  CPRB8=Main core owns pin  CPRB9=Main core owns pin  CPRB10=Main core owns pin  CPRB11=Main core owns pin  CPRB12=Main core owns pin  CPRB13=Main core owns pin  CPRB14=Main core owns pin  CPRB15=Main core owns pin  CPRC0=Main core owns pin  CPRC1=Main core owns pin  CPRC2=Main core owns pin  CPRC3=Main core owns pin  CPRC4=Main core owns pin  CPRC5=Main core owns pin  CPRC6=Main core owns pin  CPRC7=Main core owns pin  CPRC8=Main core owns pin  CPRC9=Main core owns pin  CPRC10=Main core owns pin  CPRC11=Main core owns pin  CPRC12=Main core owns pin  CPRC13=Main core owns pin  CPRC14=Main core owns pin  CPRC15=Main core owns pin  CPRD0=Main core owns pin  CPRD1=Main core owns pin  CPRD2=Main core owns pin  CPRD3=Main core owns pin  CPRD4=Main core owns pin  CPRD5=Main core owns pin  CPRD6=Main core owns pin  CPRD7=Main core owns pin  CPRD8=Main core owns pin  CPRD9=Main core owns pin  CPRD10=Main core owns pin  CPRD11=Main core owns pin  CPRD12=Main core owns pin  CPRD13=Main core owns pin  CPRD14=Main core owns pin  CPRD15=Main core owns pin  CPRE0=Main core owns pin  CPRE1=Main core owns pin  CPRE2=Main core owns pin  CPRE3=Main core owns pin  CPRE4=Main core owns pin  CPRE5=Main core owns pin  CPRE6=Main core owns pin  CPRE7=Main core owns pin  CPRE8=Main core owns pin  CPRE9=Main core owns pin  CPRE10=Main core owns pin  CPRE11=Main core owns pin  CPRE12=Main core owns pin  CPRE13=Main core owns pin  CPRE14=Main core owns pin  CPRE15=Main core owns pin  S1FNOSC=Internal Fast RC (FRC) Oscillator with postscaler  S1IESO=Start up with FRC; then switch  S1OSCIOFNC=general purpose digital I/O pin  S1FCKSM=Both Clock switching and Fail-safe Clock Monitor are disabled  S1PLLKEN=S1PLLKEN_ON  S1RWDTPS=1:1048576  S1RCLKSEL=Always use LPRC  S1WINDIS=Watchdog Timer operates in Non-Window mode  S1WDTWIN=WDT Window is 25% of WDT period  S1SWDTPS=1:1048576  S1FWDTEN=use WDTCON.ON bit  S1ICS=Communicate on PGC1 and PGD1  S1DEBUG=Not used  S1ISOLAT=The Secondary can operate (in debug mode) even if the SLVEN bit in the MSI is zero  S1NOBTSWP=BOOTSWP instruction is disabled  S1ALTI2C1=I2C1 mapped to SDA1/SCL1 pins  S1SPI1PIN=Secondary SPI1 uses I/O remap (PPS) pins  S1SSRE=Secondary generated resets will reset the Secondary Enable Bit in the MSI module  S1MSRE=The Main software oriented RESET events (RESET Op-Code; Watchdog timeout; TRAP reset; illegalInstruction) will also cause the Secondary subsystem to reset  S1CTXT1=Not Assigned  S1CTXT2=Not Assigned  S1CTXT3=Not Assigned  S1CTXT4=Not Assigned  BORLVL=BOR trip point is 2.96 V  BSSO=Normal startup operation after reset; execute instruction at 0x000000  MCA=Flash read accesses are 2 cycle to support maximum processor frequency of operation  MAXTEMP=20 ns flash access  CFGAN14=Device pin is input to AN14  CFGAN15=Device pin is input to AN15  S1IOL1WAY=Allow only one reconfiguration  S1BSSO=Normal startup operation after reset; execute instruction at 0x000000  S1BACKBUG=Not used  BISTDIS=mBIST on reset feature disabled  NOBTSWP=BOOTSWP instruction is disabled  S1BISTDIS=Secondary BIST on reset feature disabled  S1DMTIVTL=Not used  S1DMTIVTH=Not used  S1DMTCNTL=Not used  S1DMTCNTH=Not used  S1DMTDIS=Secondary Dead Man Timer is Disabled and can be enabled by software  BSEQ=Not used  IBSEQ=Not used  SMB3EN=SMBus 3.0 input levels  FUSBIDIO2=USBID pin is controlled by the USB2 module  FVBUSIO2=VBUSON pin is controlled by the USB2 module  FUSBIDIO1=USBID pin is controlled by the USB1 module  FVBUSIO1=VBUSON pin is controlled by the USB1 module  VBATBOREN=Disable ZPBOR during VBAT Mode  FDSEN=Enable DSEN bit in DSCON  BORSEL=BOR trip voltage 2.1v (Non-OPAMP deviced operation)  POSCFGAIN=Gain is G3  POSCAGCDLY=Settling time = 25ms x AGCRNG  POSCAGCRNG=Range 1x  POSCAGC=Automatic Gain Control for Oscillator  FDBGWP=Not used
      settings: SourceProductName=MPLAB Device Blocks for Simulink
  Port Info : MCHP_Blockset/System Info/Port Info  MCHP_MASTERLINK=ornek_6_2/Microchip Master
      settings: SourceProductName=MPLAB Device Blocks for Simulink
  S-R Flip-Flop : simulink_extras/Flip Flops/S-R Flip-Flop  initial_condition=0
  Scope : Scope
  wires:
  Data Type Conversion/1 -> Scope/1, Digital Output/1
  Digital Input/1 -> S-R Flip-Flop/1
  S-R Flip-Flop/1 -> Enabled Delay/2
  Enabled Delay/1 -> Data Type Conversion/1
  Constant/1 -> Enabled Delay/1
